simulink model "SH_control_harness"  (R2023b)
settings: configuration reference "ctrl_tsk_conf" (kept outside this file)
settings Model: DataDictionary=fmuGenerationDictionay.sldd  Creator=Veimar  LastModifiedBy=Veimar
settings ConfigSetRef: SourceName=ctrl_tsk_conf

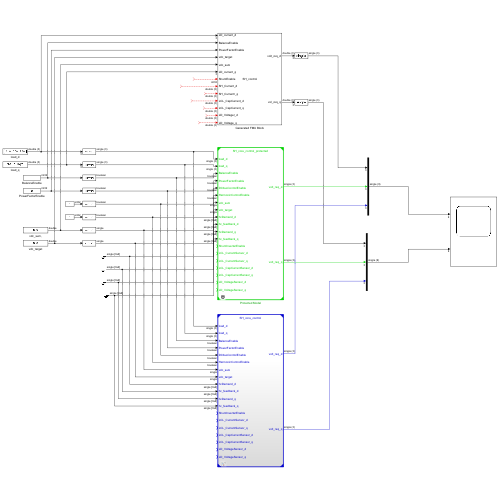
[thumbnail: Simulink's stored preview of the top-level diagram]
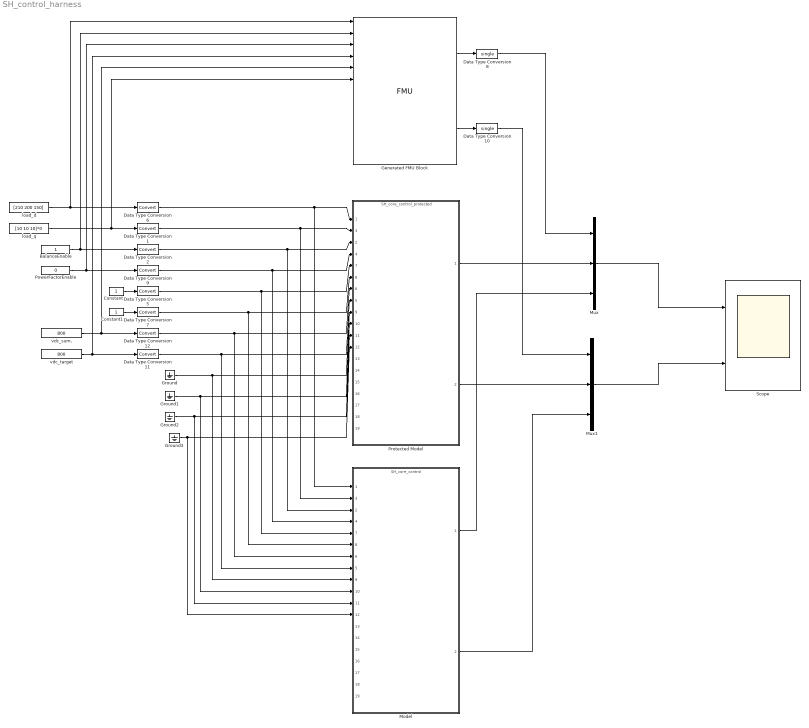
== system SH_control_harness ==
  BalanceEnable : Constant  OutDataTypeStr=int32
  Constant : Constant  OutDataTypeStr=int32
  Constant1 : Constant  OutDataTypeStr=int32
  Data Type Conversion{1..2,5..7,9,11..12} (8 alike) : DataTypeConversion  SaturateOnIntegerOverflow=off  RndMeth=Floor
  Data Type Conversion10 : DataTypeConversion  OutDataTypeStr=single  SaturateOnIntegerOverflow=off  RndMeth=Floor
  Data Type Conversion8 : DataTypeConversion  OutDataTypeStr=single  SaturateOnIntegerOverflow=off  RndMeth=Floor
  Generated FMU Block : FMU  FMUName=SH_control  FMUMode=CoSimulation  FMUSampleTime=ctrl_tsk_st  FMUCreateBusObject=off  FMUInitializeEnumObject=off  FMUCachedDialogLayout="{\"Geometry\":[1006,157,433,389],\"ParameterColumnsWidthConfig\":\"{\\\"columns\\\":[{\\\"name\\\":\\\"Parameter\\\",\\\"width\\\":145},{\\\"name\\\":\\\"Value\\\",\\\"width\\\":116},{\\\"name\\\":\\\"Unit\\\",\\\"width\\\":108},{\\\"name\\\":\\\"Description\\\",\\\"width\\\":152}]}\",\"InputColumnsWidthConfig\":[],\"OutputColumnsWidthConfig\":[]}"
      mask Type: SH_control [Co-Simulation, v2.0]
      mask Display:
      | if (exist([Simulink.fileGenControl('get','CacheFolder') '\slprj\_fmu\503b9df410b1ade17a0ae727d911ce13\SH_control\model.png'],'file'))
      |     image([Simulink.fileGenControl('get','CacheFolder') '\slprj\_fmu\503b9df410b1ade17a0ae727d911ce13\SH_control\model.png']);
      | else
      |     disp('SH_control');
      | end
      | port_label('output',1,'volt_req_d');
      | port_label('output',2,'vol_req_q');
      | port_label('input',1,'LD_current_d');
      | port_label('input',2,'BalanceEnable');
      | port_label('input',3,'PowerFactorEnable');
      | port_label('input',4,'vdc_target');
      | port_label('input',5,'vdc_sum');
      | port_label('input',6,'LD_current_q');
      | port_label('input',7,'ShuntEnable');
      | port_label('input',8,'SH_Current_d');
      | port_label('input',9,'SH_Currentr_q');
      | port_label('input',10,'LCL_CapCurrent_d');
      | port_label('input',11,'LCL_CapCurrent_q');
      | port_label('input',12,'LD_Voltager_d');
      | port_label('input',13,'LD_Voltage_q');
  Ground{,1..3} (4 alike) : Ground
  Model : ModelReference  ModelNameDialog=SH_core_control.slx  ModelReferenceVersion=1.59
      settings: PortSchema="{\"entries\":[{\"content\":{\"sides\":[{\"content\":{\"connectorIds\":[\"In1\",\"In3\",\"In2\",\"In4\",\"In7\",\"In8\",\"In6\",\"In5\",\"In9\",\"In10\",\"In11\",\"In12\",\"In13\",\"In14\",\"In15\",\"In16\",\"In17\",\"In18\",\"In19\"]},\"type\":\"ConnectorPlacement.EquallySpacedRectSide\",\"uuid\":\"23c75067-9470-41eb-93ec-30ae2c10cb0d\"},{\"content\":{\"connectorIds\":[\"Out1\",\"Out2\"],\"side\":\"RIGHT\"},\"type\":\"ConnectorPlacement.EquallySpacedRectSide\",\"uuid\":\"e9e1d1ef-f621-4d5e-b012-882bc6e1d937\"},{\"content\":{\"side\":\"TOP\"},\"type\":\"ConnectorPlacement.EquallySpacedRectSide\",\"uuid\":\"2453977c-ee77-410e-a5e8-00be7c4d652d\"}]},\"type\":\"ConnectorPlacement.EquallySpacedConnector\",\"uuid\":\"3c4f9718-bd97-403d-90d5-b0be8a0f7b23\"}],\"packageUris\":[\"http://schema.mathworks.com/mf0/Connector/R2020b\"],\"version\":\"1.0\"}"
  Mux : Mux  Inputs=3
  Mux1 : Mux  Inputs=3
  PowerFactorEnable : Constant  Value=0  OutDataTypeStr=int32
  Protected Model : ModelReference  ModelNameDialog=SH_core_control_protected.slxp  ModelReferenceVersion=1.55  CopyOfModelProtected=on
      settings: PortSchema="{\"entries\":[{\"content\":{\"sides\":[{\"content\":{\"connectorIds\":[\"In1\",\"In3\",\"In2\",\"In4\",\"In7\",\"In8\",\"In6\",\"In5\",\"In9\",\"In10\",\"In11\",\"In12\",\"In13\",\"In14\",\"In15\",\"In16\",\"In17\",\"In18\",\"In19\"]},\"type\":\"ConnectorPlacement.EquallySpacedRectSide\",\"uuid\":\"23c75067-9470-41eb-93ec-30ae2c10cb0d\"},{\"content\":{\"connectorIds\":[\"Out1\",\"Out2\"],\"side\":\"RIGHT\"},\"type\":\"ConnectorPlacement.EquallySpacedRectSide\",\"uuid\":\"e9e1d1ef-f621-4d5e-b012-882bc6e1d937\"},{\"content\":{\"side\":\"TOP\"},\"type\":\"ConnectorPlacement.EquallySpacedRectSide\",\"uuid\":\"2453977c-ee77-410e-a5e8-00be7c4d652d\"}]},\"type\":\"ConnectorPlacement.EquallySpacedConnector\",\"uuid\":\"3c4f9718-bd97-403d-90d5-b0be8a0f7b23\"}],\"packageUris\":[\"http://schema.mathworks.com/mf0/Connector/R2020b\"],\"version\":\"1.0\"}"
  Scope : Scope  NumInputPorts=2
  load_d : Constant  Value=[210 200 150]  OutDataTypeStr=double
  load_q : Constant  Value=[10 10 10]*0  OutDataTypeStr=double
  vdc_sum, : Constant  Value=800  OutDataTypeStr=double
  vdc_target : Constant  Value=800  OutDataTypeStr=double
  wires:
  Data Type Conversion5/1 -> Model/7, Protected Model/7
  PowerFactorEnable/1 -> Data Type Conversion9/1, Generated FMU Block/3
  Constant1/1 -> Data Type Conversion7/1
  Data Type Conversion11/1 -> Model/5, Protected Model/5
  Data Type Conversion7/1 -> Model/8, Protected Model/8
  Ground2/1 -> Model/11, Protected Model/11
  Data Type Conversion1/1 -> Model/3, Protected Model/3
  Ground1/1 -> Model/10, Protected Model/10
  Ground/1 -> Model/9, Protected Model/9
  Constant/1 -> Data Type Conversion5/1
  Data Type Conversion9/1 -> Model/4, Protected Model/4
  Data Type Conversion12/1 -> Model/6, Protected Model/6
  Data Type Conversion2/1 -> Model/2, Protected Model/2
  Data Type Conversion6/1 -> Model/1, Protected Model/1
  load_d/1 -> Generated FMU Block/1, Data Type Conversion6/1
  Ground3/1 -> Model/12, Protected Model/12
  BalanceEnable/1 -> Data Type Conversion2/1, Generated FMU Block/2
  load_q/1 -> Generated FMU Block/6, Data Type Conversion1/1
  Generated FMU Block/1 -> Data Type Conversion8/1
  Generated FMU Block/2 -> Data Type Conversion10/1
  vdc_sum,/1 -> Generated FMU Block/5, Data Type Conversion12/1
  vdc_target/1 -> Data Type Conversion11/1, Generated FMU Block/4
  Protected Model/1 -> Mux/2
  Protected Model/2 -> Mux1/2
  Data Type Conversion8/1 -> Mux/1
  Data Type Conversion10/1 -> Mux1/1
  Model/1 -> Mux/3
  Model/2 -> Mux1/3
  Mux/1 -> Scope/1
  Mux1/1 -> Scope/2
  ? -> Generated FMU Block/7
  ? -> Generated FMU Block/8
  ? -> Generated FMU Block/9
  ? -> Generated FMU Block/10
  ? -> Generated FMU Block/11
  ? -> Generated FMU Block/12
  ? -> Generated FMU Block/13
